simulink model "Lab2Part2"  (R2024a)
settings: Solver=VariableStepAuto  StartTime=0.0  StopTime=100  RelTol=1e-3
libraries: simulink x1
settings Model: Creator=Beast  LastModifiedBy=Beast

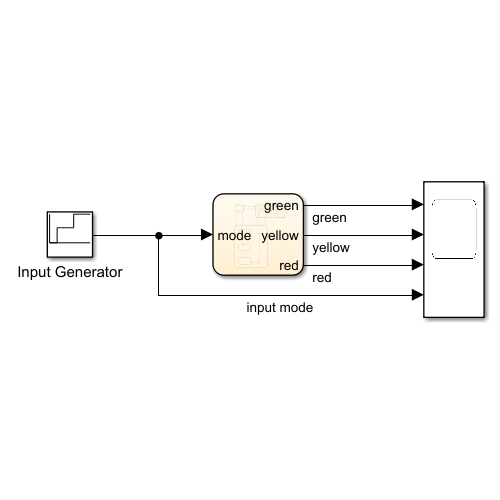
[thumbnail: Simulink's stored preview of the top-level diagram]
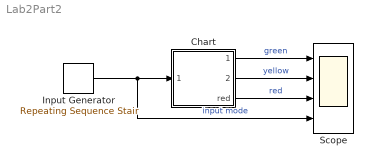
== system Lab2Part2 ==
  Chart : Stateflow chart  TreatAsAtomicUnit=on
  Input Generator : simulink/Sources/Repeating Sequence Stair  OutValues=[0 0 0 0 0 1 1 1 1 1 1 1 1 1 1 2 2 2 2 2 2 2 2 2 2].'  tsamp=-1  OutMin=[]  OutMax=[]  OutDataTypeStr=double  OutputDataTypeScalingMode=double  OutDataType=fixdt(0,8)  ConRadixGroup=Best Precision: Vector-wise  OutScaling=2^-12
      settings: LibrarySourceBlock=|
      | hdlsllib/Sources/Repeating
      | Sequence
      | Stair
  Scope : Scope  NumInputPorts=4
  wires:
  Input Generator/1 -> Scope/4, Chart/1(mode)  "input mode"
  Chart/2(yellow) -> Scope/2  "yellow"
  Chart/1(green) -> Scope/1  "green"
  Chart/3(red) -> Scope/3  "red"

== stateflow chart Lab2Part2/Chart ==
  state Off
    entry:
    green = 0;
    red = 0;
    yellow = 0;
  state Override
    state Red
      entry:
      red = 1;
      yellow = 0;
      green = 0;
    state Off
      entry:
      green = 0;
      red = 0;
      yellow = 0;
    (default) -> Override.Red
    Override.Off -> Override.Red : after(1, sec)
    Override.Red -> Override.Off : after(1, sec)
  state Normal
    state Green
      entry:
      green = 1;
      red = 0;
      yellow = 0;
    state Yellow
      entry:
      green = 0;
      red = 0;
      yellow = 1;
    state Red
      entry:
      green = 0;
      red = 1;
      yellow = 0;
    (default) -> Green
    (junction 22) -> Green
    (junction 20) -> (junction 22) : after(3, sec)
    Green -> Yellow : after(3, sec)
    Yellow -> Normal.Red : after(1, sec)
    Normal.Red -> (junction 20)
  (default) -> Off
  Off -> Override [order 1] : [mode == 2]
  Override -> Off [order 2] : [mode == 0]
  Off -> Normal [order 2] : [mode == 1]
  Normal -> Off [order 1] : [mode == 0]
  Override -> Normal [order 1] : [mode == 1]
  Normal -> Override [order 2] : [mode == 2]
  data: mode input; green output; yellow output; red output
